simulink model "Saturation_Block"  (R2022a)
settings: Solver=VariableStepAuto  StartTime=0.0  StopTime=100000  RelTol=1e-3
settings Model: Creator=maxju  LastModifiedBy=maxju

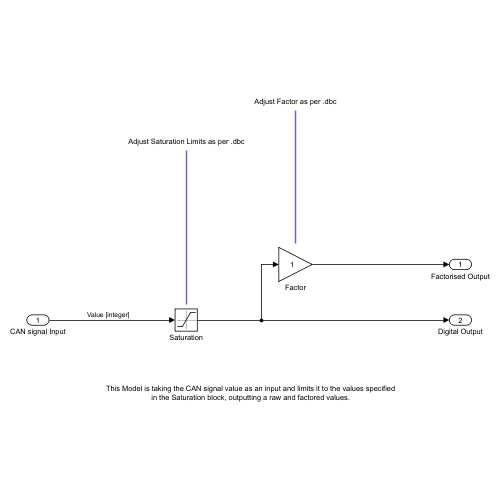
[thumbnail: Simulink's stored preview of the top-level diagram]
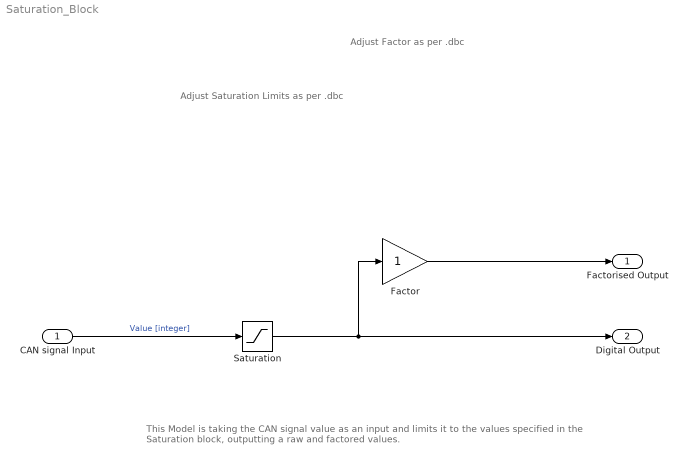
== system Saturation_Block ==
  note: Adjust Factor as per .dbc
  note: Adjust Saturation Limits as per .dbc
  note: This Model is taking the CAN signal value as an input and limits it to the values specified in the Saturation block, outputting a raw and factored values.
  CAN signal Input : Inport
  Factor : Gain  SaturateOnIntegerOverflow=on  OutDataTypeStr=Inherit: Same as input  ParamDataTypeStr=Inherit: Same as input
  Saturation : Saturate  UpperLimit=100  LowerLimit=-100
  Factorised Output : Outport
  Digital Output : Outport  Port=2
  wires:
  Saturation/1 -> Digital Output/1, Factor/1
  CAN signal Input/1 -> Saturation/1  "Value [integer]"
  Factor/1 -> Factorised Output/1
